simulink model "susp_vehi"  (R2018a)
settings: Solver=VariableStepAuto  StartTime=0.0  StopTime=3  RelTol=1e-3
InitFcn:
  | sis_sus_vehiculo
values from neighbouring files (symbols this model uses):
  b = 40    [sis_sus_vehiculo.m]
  k1 = 10000    [sis_sus_vehiculo.m]
  k2 = 2000    [sis_sus_vehiculo.m]
  m1 = 10    [sis_sus_vehiculo.m]
  m2 = 3000    [sis_sus_vehiculo.m]
settings Model: Creator=cmparedes  LastModifiedBy=carma

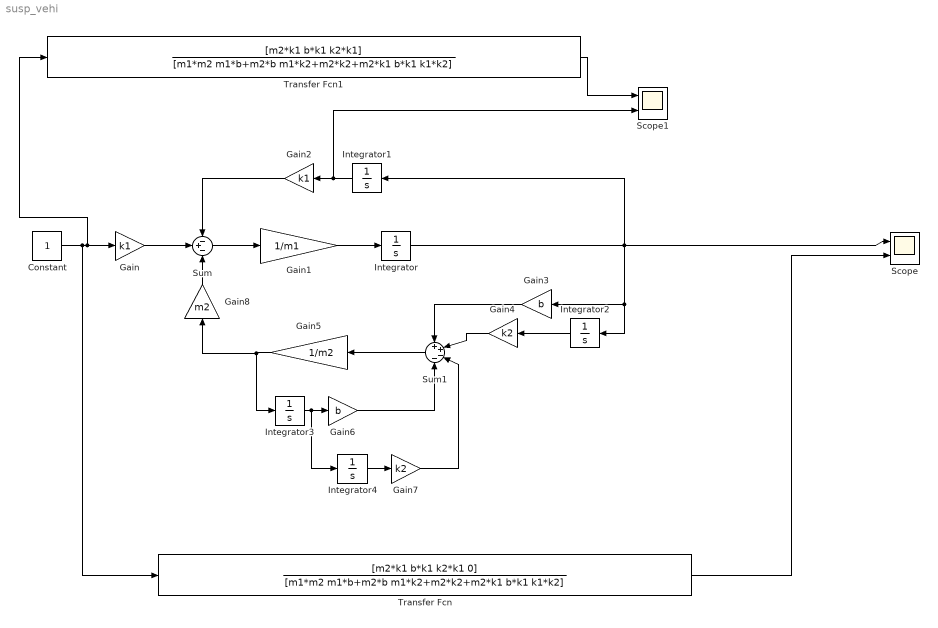
== system susp_vehi ==
  Constant : Constant
  Gain : Gain  Gain=k1
  Gain1 : Gain  Gain=1/m1
  Gain2 : Gain  Gain=k1
  Gain3 : Gain  Gain=b
  Gain4 : Gain  Gain=k2
  Gain5 : Gain  Gain=1/m2
  Gain6 : Gain  Gain=b
  Gain7 : Gain  Gain=k2
  Gain8 : Gain  Gain=m2
  Integrator{,1..4} (5 alike) : Integrator
  Scope : Scope  NumInputPorts=2
  Scope1 : Scope  NumInputPorts=2
  Sum : Sum  Inputs=-+-
  Sum1 : Sum  Inputs=++--
  Transfer Fcn : TransferFcn  Numerator=[m2*k1 b*k1 k2*k1 0]  Denominator=[m1*m2 m1*b+m2*b m1*k2+m2*k2+m2*k1 b*k1 k1*k2]
  Transfer Fcn1 : TransferFcn  Numerator=[m2*k1 b*k1 k2*k1]  Denominator=[m1*m2 m1*b+m2*b m1*k2+m2*k2+m2*k1 b*k1 k1*k2]
  wires:
  Gain/1 -> Sum/2
  Sum/1 -> Gain1/1
  Gain1/1 -> Integrator/1
  Integrator1/1 -> Scope1/2, Gain2/1
  Gain2/1 -> Sum/1
  Integrator/1 -> Integrator2/1, Gain3/1, Scope/1, Integrator1/1
  Gain3/1 -> Sum1/1
  Integrator2/1 -> Gain4/1
  Gain4/1 -> Sum1/2
  Sum1/1 -> Gain5/1
  Gain5/1 -> Gain8/1, Integrator3/1
  Integrator3/1 -> Integrator4/1, Gain6/1
  Gain6/1 -> Sum1/4
  Integrator4/1 -> Gain7/1
  Gain7/1 -> Sum1/3
  Gain8/1 -> Sum/3
  Transfer Fcn/1 -> Scope/2
  Transfer Fcn1/1 -> Scope1/1
  Constant/1 -> Transfer Fcn/1, Transfer Fcn1/1, Gain/1
